simulink model "thruster"  (R2025b)
settings: Solver=VariableStepAuto  StartTime=0.0  StopTime=30  FixedStep=0.1  RelTol=1e-3
libraries: simulink x1, slpidlib x1
settings Model: Creator=wangzerun  LastModifiedBy=wangzerun

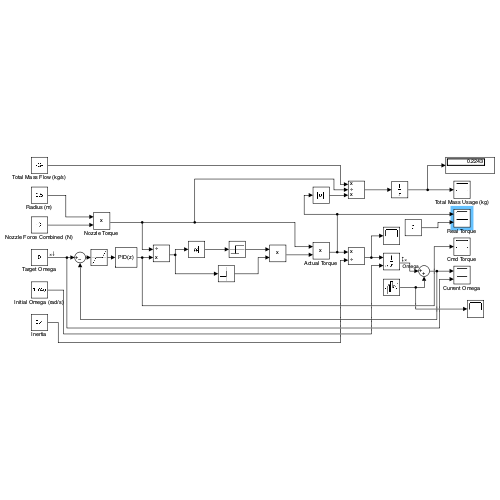
[thumbnail: Simulink's stored preview of the top-level diagram]
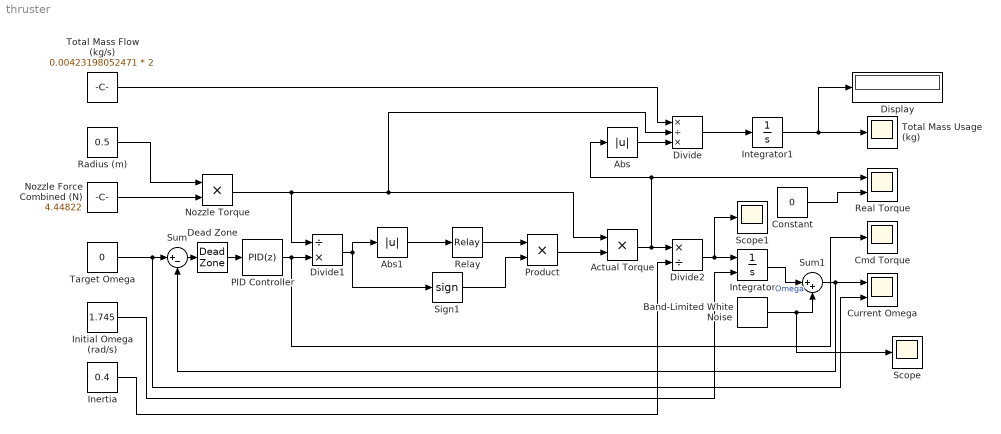
== system thruster ==
  Abs : Abs  ZeroCross=off  SaturateOnIntegerOverflow=off
  Abs1 : Abs  SaturateOnIntegerOverflow=off
  Actual Torque : Product
  Band-Limited White Noise : simulink/Sources/Band-Limited White Noise  Cov=(30 * pi/180)^2 * 2  Ts=2  seed=[23341]
  Cmd Torque : Scope
      settings: ActiveDisplayYMinimum=-7.1662592998233725  ActiveDisplayYMaximum=6.9961529161590548  DataLoggingVariableName=ScopeData3
  Constant : Constant  Value=0
  Current Omega : Scope  NumInputPorts=2
      settings: ActiveDisplayYMinimum=-2.5365872632183852  ActiveDisplayYMaximum=2.4281460211817203
  Dead Zone : DeadZone  LowerValue=-0.015  UpperValue=0.015
  Display : Display
  Divide : Product  Inputs=*/*
  Divide1 : Product  Inputs=/*
  Divide2 : Product  Inputs=*/
  Inertia : Constant  Value=0.4
  Initial Omega (rad/s) : Constant  Value=1.745
  Integrator : Integrator  InitialConditionSource=external  InitialCondition=10
  Integrator1 : Integrator
  Nozzle Force Combined (N) : Constant  Value=4.44822
  Nozzle Torque : Product
  PID Controller : slpidlib/PID Controller  Controller=PID  Form=Parallel  TimeDomain=Discrete-time  UseExternalTs=off  SampleTime=0.1  IntegratorMethod=Forward Euler  FilterMethod=Forward Euler  ControllerParametersSource=internal  P=2  I=1.3  UseKiTs=off  D=2  UseExternalDerivativeSource=off  N=0.5  UseFilter=on  TunerSelectOption=Transfer Function Based (PID Tuner App)  InitialConditionSource=internal  InitialConditionForIntegrator=0  InitialConditionForFilter=0  DifferentiatorICPrevScaledInput=0  ExternalReset=none  TrackingMode=off  Kt=1  LimitOutput=off  SatLimitsSource=internal  UpperSaturationLimit=inf  LowerSaturationLimit=-inf  LinearizeAsGain=on  AntiWindupMode=none  Kb=1  LimitIntegrator=off  UpperIntegratorSaturationLimit=inf  LowerIntegratorSaturationLimit=-inf  POutMin=[]  POutMax=[]  IOutMin=[]  IOutMax=[]  DOutMin=[]  DOutMax=[]  NOutMin=[]  NOutMax=[]  SumOutMin=[]  SumOutMax=[]  SaturationOutMin=[]  SaturationOutMax=[]  PParamMin=[]  PParamMax=[]  IParamMin=[]  IParamMax=[]  DParamMin=[]  DParamMax=[]  NParamMin=[]  NParamMax=[]  KbParamMin=[]  KbParamMax=[]  KtParamMin=[]  KtParamMax=[]  KbOutMin=[]  KbOutMax=[]  KtOutMin=[]  KtOutMax=[]  IntegratorOutMin=[]  IntegratorOutMax=[]  FilterOutMin=[]  FilterOutMax=[]  SumI1OutMin=[]  SumI1OutMax=[]  SumI2OutMin=[]  SumI2OutMax=[]  SumI3OutMin=[]  SumI3OutMax=[]  SumI4OutMin=[]  SumI4OutMax=[]  SumDOutMin=[]  SumDOutMax=[]  DifferentiatorOutMin=[]  DifferentiatorOutMax=[]  FilterDiffOutCoefMin=[]  FilterDiffOutCoefMax=[]  ReciprocalOutMin=[]  ReciprocalOutMax=[]  SumDenOutMin=[]  SumDenOutMax=[]  SumNumOutMin=[]  SumNumOutMax=[]  DivideOutMin=[]  DivideOutMax=[]  UdiffTsProdOutMin=[]  UdiffTsProdOutMax=[]  NTsProdOutMin=[]  NTsProdOutMax=[]  UintegralTsProdOutMin=[]  UintegralTsProdOutMax=[]  UngainTsProdOutMin=[]  UngainTsProdOutMax=[]  ClampingZeroOutDataTypeStr=Inherit: Inherit via back propagation  ClampingZeroOutMin=[]  ClampingZeroOutMax=[]  FilterDenConstantOutDataTypeStr=Inherit: Inherit via back propagation  FilterDenConstantOutMin=[]  FilterDenConstantOutMax=[]  PCopyOutDataTypeStr=Inherit: Inherit via back propagation  PCopyOutMin=[]  PCopyOutMax=[]  NCopyOutDataTypeStr=Inherit: Inherit via back propagation  NCopyOutMin=[]  NCopyOutMax=[]  IntegratorContinuousStateAttributes=''  IntegratorStateMustResolveToSignalObject=off  IntegratorRTWStateStorageClass=Auto  FilterContinuousStateAttributes=''  FilterStateMustResolveToSignalObject=off  FilterRTWStateStorageClass=Auto  ParallelPVariant=InternalParameters  IdealPVariant=Disabled  IVariant=InternalParameters  DVariant=InternalParameters  IntegratorVariant=Discrete  SatVariant=Disabled  AWVariant=Passthrough  PCopyVariant=Disabled  TRVariant=Disabled  FdbkBlocksVariant=Forward  IdealPFdbkVariant=Disabled  SatFdbkVariant=Disabled  DerivativeFilterVariant=ForwardEulerFilter  NVariant=InternalParameters  NCopyVariant=Disabled  FilterICVariant=InternalICsFilter  IntegratorICVariant=InternalICs  ExternalResetVariant=Disabled  TRSumVariant=Passthrough  SumFdbkVariant=Disabled  SumVariant=Sum_PID  TsampFilterVariant=InternalTs  TsampNgainVariant=Passthrough  TsampIntegralVariant=Disabled_SignalSpec  ExternalSaturationOutDataTypeStr=Inherit: Same as second input  DerivativeSourceVariant=ErrorSignal  PreIntVariant=InternalPreInt
  Product : Product
  Radius (m) : Constant  Value=0.5
  Real Torque : Scope  NumInputPorts=2
      settings: ActiveDisplayYMinimum=-2.7801375  ActiveDisplayYMaximum=2.7801375  DataLoggingVariableName=ScopeData2
  Relay : Relay  OnSwitchValue=0.1  OffSwitchValue=0.1
  Scope : Scope
      settings: ActiveDisplayYMinimum=-1  ActiveDisplayYMaximum=1  DataLoggingVariableName=ScopeData4
  Scope1 : Scope
      settings: ActiveDisplayYMinimum=-1  ActiveDisplayYMaximum=1  DataLoggingVariableName=ScopeData5
  Sign1 : Signum  ZeroCross=off
  Sum : Sum  Inputs=|+-
  Sum1 : Sum  Inputs=|++
  Target Omega : Constant  Value=0
  Total Mass Flow (kg/s) : Constant  Value=0.00423198052471 * 2
  Total Mass Usage (kg) : Scope
      settings: ActiveDisplayYMinimum=-0.0022217897754727607  ActiveDisplayYMaximum=0.01999610797925485
  wires:
  Target Omega/1 -> Current Omega/2, Sum/1
  Nozzle Force Combined (N)/1 -> Nozzle Torque/2
  Nozzle Torque/1 -> Divide1/1, Divide/2, Actual Torque/1
  Abs/1 -> Divide/3
  Radius (m)/1 -> Nozzle Torque/1
  Total Mass Flow (kg/s)/1 -> Divide/1
  Divide/1 -> Integrator1/1
  Integrator1/1 -> Display/1, Total Mass Usage (kg)/1
  Actual Torque/1 -> Abs/1, Real Torque/1, Divide2/1
  Initial Omega (rad/s)/1 -> Integrator/2
  Divide2/1 -> Scope1/1, Integrator/1
  Inertia/1 -> Divide2/2
  PID Controller/1 -> Divide1/2, Cmd Torque/1
  Constant/1 -> Real Torque/2
  Product/1 -> Actual Torque/2
  Divide1/1 -> Abs1/1, Sign1/1
  Sum/1 -> Dead Zone/1
  Dead Zone/1 -> PID Controller/1
  Sum1/1 -> Sum/2, Current Omega/1
  Integrator/1 -> Sum1/1  "Omega"
  Band-Limited White Noise/1 -> Sum1/2, Scope/1
  Relay/1 -> Product/1
  Abs1/1 -> Relay/1
  Sign1/1 -> Product/2
